simulink model "sim_ip_servo"  (R2023a)
settings: Solver=ode4  StartTime=0.0  StopTime=inf  FixedStep=0.001  RelTol=1e-3
values from neighbouring files (symbols this model uses):
  alpha1 = 2.42e-01    (= 0.242)    [ip_servo_design.m]
  alpha2 = 1.17e-01    (= 0.117)    [ip_servo_design.m]
  delta1 = 1.51e+00    (= 1.51)    [ip_servo_design.m]
  G = Ke(5)    [ip_servo_design.m]
  g = 9.81e+00    (= 9.81)    [ip_servo_design.m]
  K = Ke(1:4)    [ip_servo_design.m]
  L1 = 1.02e-01    (= 0.102)    [ip_servo_design.m]
  mu1 = 9.67e-01    (= 0.967)    [ip_servo_design.m]
  mu2 = 4.24e-02    (= 0.0424)    [ip_servo_design.m]
  Tf1 = 0.05    [ip_servo_design.m]
  Tf2 = 0.05    [ip_servo_design.m]
undefined symbols (not defined in the file or in its folder): sgn
settings Model: PacingRate=5  Creator=kawata  LastModifiedBy=kawata
settings DataIOCC: ReturnWorkspaceOutputs=off
settings RTWCC: GPUComputeCapability=5.0

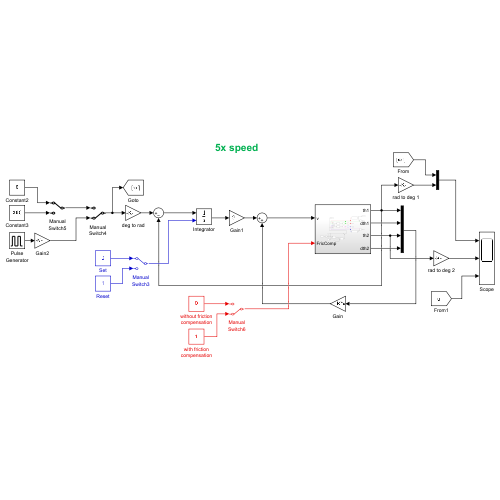
[thumbnail: Simulink's stored preview of the top-level diagram]
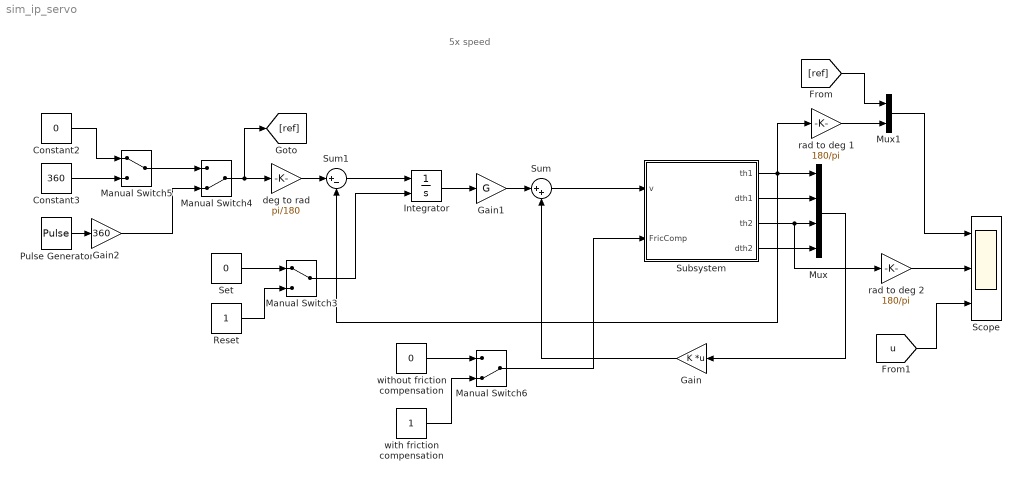
== system sim_ip_servo ==
  note: 5x speed
  Constant2 : Constant  Value=0
  Constant3 : Constant  Value=360
  Gain : Gain  Gain=K  Multiplication=Matrix(K*u)
  Gain1 : Gain  Gain=G
  Gain2 : Gain  Gain=360
  Integrator : Integrator  ExternalReset=level hold
  Manual Switch3 : ManualSwitch
  Manual Switch4 : ManualSwitch  CurrentSetting=0
  Manual Switch5 : ManualSwitch
  Manual Switch6 : ManualSwitch  CurrentSetting=0
  Mux : Mux
  Mux1 : Mux  Inputs=2
  Pulse Generator : DiscretePulseGenerator  PulseType=Time based  Period=16  PulseWidth=50  PhaseDelay=4
  Reset : Constant
  Scope : Scope  NumInputPorts=3
  Set : Constant  Value=0
  Subsystem : Subsystem
  Sum : Sum  Inputs=|++
  Sum1 : Sum  Inputs=|+-
  deg to rad : Gain  Gain=pi/180
  rad to deg 1 : Gain  Gain=180/pi
  rad to deg 2 : Gain  Gain=180/pi
  with friction compensation : Constant
  without friction compensation : Constant  Value=0
  wires:
  Mux1/1 -> Scope/1
  Manual Switch6/1 -> Subsystem/2(FricComp)
  without friction compensation/1 -> Manual Switch6/1
  with friction compensation/1 -> Manual Switch6/2
  Manual Switch4/1 -> [ref], deg to rad/1
  rad to deg 2/1 -> Scope/2
  Sum/1 -> Subsystem/1(v)
  Set/1 -> Manual Switch3/1
  Reset/1 -> Manual Switch3/2
  Pulse Generator/1 -> Gain2/1
  Gain1/1 -> Sum/1
  Gain2/1 -> Manual Switch4/2
  Constant3/1 -> Manual Switch5/2
  deg to rad/1 -> Sum1/1
  Mux/1 -> Gain/1
  Constant2/1 -> Manual Switch5/1
  Subsystem/2(dth1) -> Mux/2
  Manual Switch5/1 -> Manual Switch4/1
  Gain/1 -> Sum/2
  Sum1/1 -> Integrator/1
  [ref] -> Mux1/1
  rad to deg 1/1 -> Mux1/2
  Subsystem/4(dth2) -> Mux/4
  Manual Switch3/1 -> Integrator/2
  Subsystem/1(th1) -> Mux/1, rad to deg 1/1, Sum1/2
  Integrator/1 -> Gain1/1
  Subsystem/3(th2) -> Mux/3, rad to deg 2/1
  [u] -> Scope/3

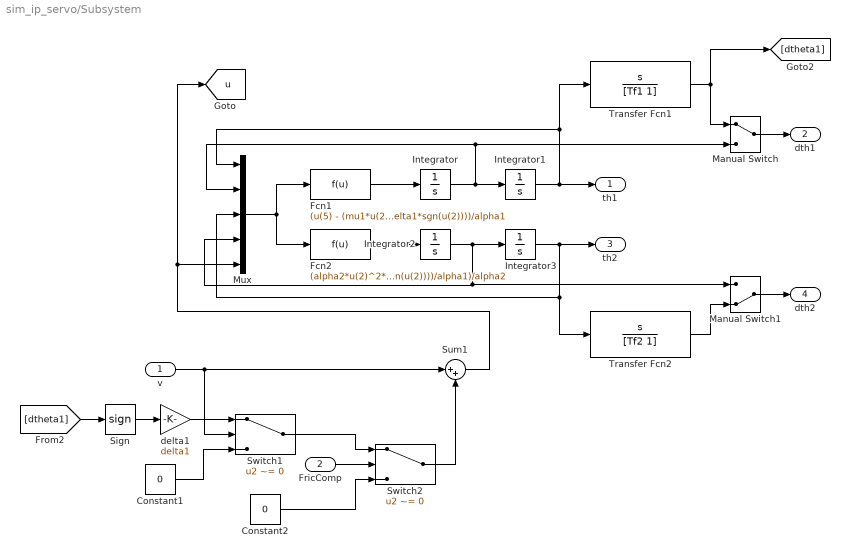
== system sim_ip_servo/Subsystem ==
  v : Inport
  FricComp : Inport  Port=2
  Constant1 : Constant  Value=0
  Constant2 : Constant  Value=0
  Fcn1 : Fcn  Expr=(u(5) - (mu1*u(2) + delta1*sgn(u(2))))/alpha1
  Fcn2 : Fcn  Expr=(alpha2*u(2)^2*sin(u(3))*cos(u(3)) + g*sin(u(3)) - mu2*u(4) - L1*cos(u(3))*(u(5) - (mu1*u(2) + delta1*sgn(u(2))))/alpha1)/alpha2
  Integrator{,1..3} (4 alike) : Integrator
  Manual Switch : ManualSwitch
  Manual Switch1 : ManualSwitch  CurrentSetting=0
  Mux : Mux  Inputs=5
  Sign : Signum
  Sum1 : Sum  Inputs=|++
  Switch1 : Switch  Criteria=u2 ~= 0  SaturateOnIntegerOverflow=off  InputSameDT=off
  Switch2 : Switch  Criteria=u2 ~= 0  SaturateOnIntegerOverflow=off  InputSameDT=off
  Transfer Fcn1 : TransferFcn  Numerator=[1 0]  Denominator=[Tf1 1]
  Transfer Fcn2 : TransferFcn  Numerator=[1 0]  Denominator=[Tf2 1]
  delta1 : Gain  Gain=delta1
  th1 : Outport
  dth1 : Outport  Port=2
  th2 : Outport  Port=3
  dth2 : Outport  Port=4
  tag scope: u=global
  wires:
  Integrator3/1 -> th2/1, Transfer Fcn2/1, Mux/3
  Fcn1/1 -> Integrator/1
  Fcn2/1 -> Integrator2/1
  Mux/1 -> Fcn2/1, Fcn1/1
  Integrator1/1 -> Transfer Fcn1/1, Mux/1, th1/1
  Integrator/1 -> Mux/2, Manual Switch/2, Integrator1/1
  Integrator2/1 -> Mux/4, Manual Switch1/1, Integrator3/1
  Manual Switch/1 -> dth1/1
  Manual Switch1/1 -> dth2/1
  Transfer Fcn1/1 -> [dtheta1], Manual Switch/1
  Transfer Fcn2/1 -> Manual Switch1/2
  Sum1/1 -> [u], Mux/5
  Constant2/1 -> Switch2/3
  Switch1/1 -> Switch2/1
  [dtheta1] -> Sign/1
  Switch2/1 -> Sum1/2
  Sign/1 -> delta1/1
  v/1 -> Switch1/2, Sum1/1
  Constant1/1 -> Switch1/3
  FricComp/1 -> Switch2/2
  delta1/1 -> Switch1/1
